simulink library "stm32f4_io_lib"  (R2015b)
settings: Solver=ode45  StartTime=0.0  StopTime=10.0  RelTol=1e-3
libraries: simulink x9
settings Model: Creator=Krisada  LastModifiedBy=Aimagin
settings DataIOCC: SaveFormat=Array  SignalLoggingSaveFormat=ModelDataLogs
settings OptimizationCC: ExpressionDepthLimit=2147483647
settings DebuggingCC: UnderspecifiedInitializationDetection=Classic  MergeDetectMultiDrivingBlocksExec=none  SolverPrmCheckMsg=warning  FcnCallInpInsideContextMsg=UseLocalSettings  StateNameClashWarn=warning  StrictBusMsg=Warning
settings HardwareCC: ProdBitPerPointer=32  ProdLargestAtomicFloat=None  ProdIntDivRoundTo=Undefined  ProdEndianess=Unspecified  ProdWordSize=32  ProdHWDeviceType=32-bit Generic
settings GRTTargetCC: CombineOutputUpdateFcns=off  GRTInterface=on
settings ConfigComp: CovModelRefEnable=Off

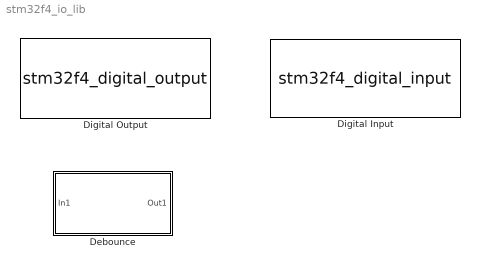
== system stm32f4_io_lib ==
  Debounce : Subsystem  TreatAsAtomicUnit=on  mask{mode=Normal, prescale=4, debounce=4}
      mask prompts: prescale "Prescale (Debounce count)"; debounce "Debounce value"
      mask help:
      | Mode,
      | 1. Normal:
      |  - Output state is 0 (FALSE) when input is steady at 0 for a Debounce period (or longer).
      |  - Output state is 1 (TRUE) when input is steady at non-zero for a Debounce period (or longer).
      |
      | 2. Single Pulse:
      |  - Output state will generate a single pulse (one time-step) when input signal change from 0-to-NonZero and steady for a Debounce period.
      |
      | 3. Toggle Latch:
      |  - Output state will toggle when input signal change from 0-to-NonZero and steady for a Debounce period
      |
      | Debounce period,
      |  - Debounce period (sec) = Debounce count * Sample time (sec)
      |
      | Note: the block is Masked Subsystem, to see its function: from the popup menu on mouse right-click, select "Look Under Mask".
      settings: RTWFcnNameOpts=Use subsystem name  RTWFileNameOpts=Use function name
      mask Help: web(fullfile(waijungdocroot,'gpio_debounce.htm'),'-browser')
      mask TypeOptions mode: Normal | Single Pulse | Toggle Latch
      mask Callback mode: waijung_intput_validation_callback('mode');
      mask TypeOptions prescale: 4 | 8 | 16 | 32 | 64 | 128 | 256 | 512 | 1024 | 2048 | 4096 | 8192
      mask Callback debounce: waijung_intput_validation_callback('prescale');
      mask Display: disp('Button Pressed\n(Normal)\nDebounce count: 4');
  Digital Input : S-Function  FunctionName=stm32f4_digital_input  Parameters=port,speed,porttype,porttypestr,use_pin0,use_pin1,use_pin2,use_pin3,use_pin4,use_pin5,use_pin6,use_pin7,use_pin8,use_pin9,use_pin10,use_pin11,use_pin12,use_pin13,use_pin14,use_pin15,pinstr,usedpinarray,bitbandingstr,sampletime,sampletimestr,blockid,glabalinit  SFunctionDeploymentMode=off  EnableBusSupport=off  mask(stm32f4_digital_input){port=A, speed=100, porttype=None, porttypestr=NOPULL, use_pin0=on, use_pin1=on, use_pin2=off, use_pin3=off, use_pin4=off, use_pin5=off, use_pin6=off, use_pin7=off, use_pin8=off, use_pin9=off, use_pin10=off, use_pin11=off, use_pin12=off, use_pin13=off, use_pin14=off, use_pin15=off, pinstr=GPIO_Pin_0 | GPIO_Pin_1, usedpinarray=[1  1  0  0  0  0  0  0  0  0  0  0  0  0  0  0], bitbandingstr=|, sampletime=-1, sampletimestr=0, blockid=DigitalInput, enablecustomportlabel=off, glabalinit=off, cinputportlabel=In1, In2, coutputportlabel=Out1, Out2}
      mask bitbandingstr=|
      | #define DigitalInput_A0 Peripheral_BB(GPIOA->IDR, 0)  /* Output pin */
      | #define DigitalInput_A1 Peripheral_BB(GPIOA->IDR, 1)  /* Output pin */
      mask prompts: speed "Speed (MHz)"; porttype "Type (Pull-Up/Pull-Down)"; porttypestr "Type (Pull Up/Pull Down) String"; use_pin0 "Use Pin 0"; use_pin1 "Use Pin 1"; use_pin2 "Use Pin 2"; use_pin3 "Use Pin 3"; use_pin4 "Use Pin 4"; use_pin5 "Use Pin 5"; use_pin6 "Use Pin 6"; use_pin7 "Use Pin 7"; use_pin8 "Use Pin 8"; use_pin9 "Use Pin 9"; use_pin10 "Use Pin 10"; use_pin11 "Use Pin 11"; use_pin12 "Use Pin 12"; use_pin13 "Use Pin 13"; use_pin14 "Use Pin 14"; use_pin15 "Use Pin 15"; pinstr "Pin string"; usedpinarray "Used pin array"; bitbandingstr "Bit banding string"; sampletime "Sample time (sec)"; sampletimestr "Compiled sample time (sec) in string"; enablecustomportlabel "Enable custom port labels"; glabalinit "Use global initialization"; cinputportlabel "Custom input port labels (Ex. In1, In2, In3)"; coutputportlabel "Custom output port labels (Ex. Out1, Out2, Out3)"
      mask help: This block implements Digital Input Module.
      mask init:
      | stm32f4_digital_input_callback('init');
      mask Help: web(fullfile(waijungdocroot,'stm32f4_digital_input.htm'), '-browser')
      mask TypeOptions port: A | B | C | D | E | F | G | H | I | J | K
      mask Callback port: stm32f4_digital_input_callback('port');
      mask TypeOptions speed: 2 | 25 | 50 | 100
      mask Callback speed: stm32f4_digital_input_callback('speed');
      mask TypeOptions porttype: None | Pull Up | Pull Down
      mask Callback porttype: stm32f4_digital_input_callback('porttype');
      mask Callback porttypestr: stm32f4_digital_input_callback('porttypestr');
      mask Callback pinstr: stm32f4_digital_input_callback('pinstr');
      mask Callback usedpinarray: stm32f4_digital_input_callback('usedpinarray');
      mask Callback bitbandingstr: stm32f4_digital_input_callback('bitbandingstr');
      mask Callback sampletime: stm32f4_digital_input_callback('sampletime');
      mask Callback sampletimestr: stm32f4_digital_input_callback('sampletimestr');
      mask Callback blockid: stm32f4_digital_input_callback('blockid');
      mask Callback enablecustomportlabel: stm32f4_digital_input_callback('enablecustomportlabel');
      mask Display: text(0.05, 0.5, 'Port: A\nSpeed (MHz): 100\nType (PU/PD): None\nTs (sec): 0','ver','middle','hor','left');port_label('output', 1,'PA0');port_label('output', 2,'PA1')
  Digital Output : S-Function  FunctionName=stm32f4_digital_output  Parameters=use_bitband,port,speed,porttype,porttypestr,use_pin0,use_pin1,use_pin2,use_pin3,use_pin4,use_pin5,use_pin6,use_pin7,use_pin8,use_pin9,use_pin10,use_pin11,use_pin12,use_pin13,use_pin14,use_pin15,pinstr,usedpinarray,bitbandingstr,sampletime,sampletimestr,blockid,globalinit  SFunctionDeploymentMode=off  EnableBusSupport=off  mask(stm32f4_digital_output){use_bitband=on, port=D, speed=100, porttype=Push Pull, porttypestr=PP, use_pin0=off, use_pin1=off, use_pin2=off, use_pin3=off, use_pin4=off, use_pin5=off, use_pin6=off, use_pin7=off, use_pin8=off, use_pin9=off, use_pin10=off, use_pin11=off, use_pin12=on, use_pin13=on, use_pin14=on, use_pin15=on, pinstr=GPIO_Pin_12 | GPIO_Pin_13 | GPIO_Pin_14 | GPIO_Pin_15, usedpinarray=[0  0  0  0  0  0  0  0  0  0  0  0  1  1  1  1], bitbandingstr=|, sampletime=-1, sampletimestr=0, blockid=DigitalOutput, enablecustomportlabel=off, globalinit=off, cinputportlabel=In1, In2, coutputportlabel=0}
      mask bitbandingstr=|
      | #define DigitalOutput_D12 Peripheral_BB(GPIOD->ODR, 12)  /* Output pin */
      | #define DigitalOutput_D13 Peripheral_BB(GPIOD->ODR, 13)  /* Output pin */
      | #define DigitalOutput_D14 Peripheral_BB(GPIOD->ODR, 14)  /* Output pin */
      | #define DigitalOutput_D15 Peripheral_BB(GPIOD->ODR, 15)  /* Output pin */
      mask prompts: use_bitband "Use Bit banding"; speed "Speed (MHz)"; porttype "Type (Push-Pull/Open-Drain)"; porttypestr "Type (Push-Pull/Open-Drain) String"; use_pin0 "Use Pin 0"; use_pin1 "Use Pin 1"; use_pin2 "Use Pin 2"; use_pin3 "Use Pin 3"; use_pin4 "Use Pin 4"; use_pin5 "Use Pin 5"; use_pin6 "Use Pin 6"; use_pin7 "Use Pin 7"; use_pin8 "Use Pin 8"; use_pin9 "Use Pin 9"; use_pin10 "Use Pin 10"; use_pin11 "Use Pin 11"; use_pin12 "Use Pin 12"; use_pin13 "Use Pin 13"; use_pin14 "Use Pin 14"; use_pin15 "Use Pin 15"; pinstr "Pin string"; usedpinarray "Used pin array"; bitbandingstr "Bit banding string"; sampletime "Sample time (sec)"; sampletimestr "Compiled sample time (sec) in string"; enablecustomportlabel "Enable custom port labels"; globalinit "Use global initialization"; cinputportlabel "Custom input port labels (Ex. In1, In2, In3)"; coutputportlabel "Custom output port labels (Ex. Out1, Out2, Out3)"
      mask help: This block implements Digital Output Module.
      mask init:
      | stm32f4_digital_output_callback('init');
      mask Help: web(fullfile(waijungdocroot,'stm32f4_digital_output.htm'),'-browser')
      mask TypeOptions port: A | B | C | D | E | F | G | H | I | J | K
      mask Callback port: stm32f4_digital_output_callback('port');
      mask TypeOptions speed: 2 | 25 | 50 | 100
      mask Callback speed: stm32f4_digital_output_callback('speed');
      mask TypeOptions porttype: Push Pull | Open Drain
      mask Callback porttype: stm32f4_digital_output_callback('porttype');
      mask Callback porttypestr: stm32f4_digital_output_callback('porttypestr');
      mask Callback pinstr: stm32f4_digital_output_callback('pinstr');
      mask Callback usedpinarray: stm32f4_digital_output_callback('usedpinarray');
      mask Callback bitbandingstr: stm32f4_digital_output_callback('bitbandingstr');
      mask Callback sampletime: stm32f4_digital_output_callback('sampletime');
      mask Callback sampletimestr: stm32f4_digital_output_callback('sampletimestr');
      mask Callback blockid: stm32f4_digital_output_callback('blockid');
      mask Callback enablecustomportlabel: stm32f4_digital_output_callback('enablecustomportlabel');
      mask Display: text(0.95, 0.5, 'Port: D\nSpeed (MHz): 100\nType (PP/OD): Push Pull\nTs (sec): 0','ver','middle','hor','right');port_label('input', 1,'PD12');port_label('input', 2,'PD13');port_label('input', 3,'PD14');port_label('input', 4,'PD15')

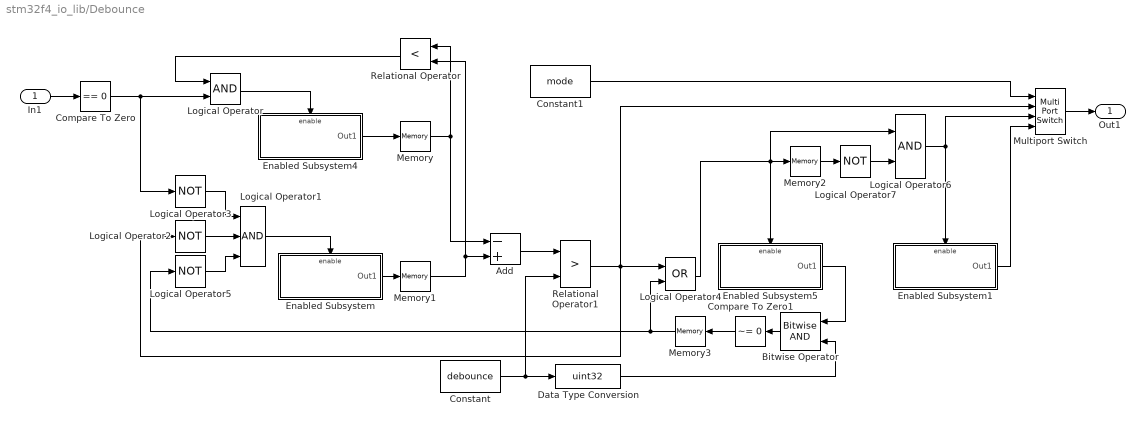
== system stm32f4_io_lib/Debounce ==
  In1 : Inport
  Add : Sum  Inputs=-+  OutDataTypeStr=int32
  Bitwise Operator : simulink/Logic and Bit Operations/Bitwise Operator  logicop=AND  UseBitMask=off  NumInputPorts=2  BitMask=debouce  BitMaskRealWorld=Stored Integer
  Compare To Zero : simulink/Logic and Bit Operations/Compare To Zero  SystemSampleTime=-1  relop===  LogicOutDataTypeMode=uint8  ZeroCross=off
  Compare To Zero1 : simulink/Logic and Bit Operations/Compare To Zero  SystemSampleTime=-1  relop=~=  LogicOutDataTypeMode=boolean  ZeroCross=off
  Constant : Constant  Value=debounce  OutDataTypeStr=int32  SampleTime=-1
  Constant1 : Constant  Value=mode  OutDataTypeStr=int32  SampleTime=-1
  Data Type Conversion : DataTypeConversion  OutDataTypeStr=uint32
  Enabled Subsystem : Subsystem  TreatAsAtomicUnit=on
  Enabled Subsystem1 : Subsystem  TreatAsAtomicUnit=on
  Enabled Subsystem4 : Subsystem  TreatAsAtomicUnit=on
  Enabled Subsystem5 : Subsystem  TreatAsAtomicUnit=on
  Logical Operator : Logic  AllPortsSameDT=off  OutDataTypeStr=boolean
  Logical Operator1 : Logic  Inputs=3  AllPortsSameDT=off  OutDataTypeStr=boolean
  Logical Operator{2..3,5,7} (4 alike) : Logic  Operator=NOT  AllPortsSameDT=off  OutDataTypeStr=boolean
  Logical Operator4 : Logic  Operator=OR  AllPortsSameDT=off  OutDataTypeStr=boolean
  Logical Operator6 : Logic  AllPortsSameDT=off  OutDataTypeStr=boolean
  Memory{,1..3} (4 alike) : Memory  InheritSampleTime=on  LinearizeMemory=on  LinearizeAsDelay=on
  Multiport Switch : MultiPortSwitch
  Relational Operator : RelationalOperator  Operator=<  OutDataTypeStr=boolean
  Relational Operator1 : RelationalOperator  Operator=>  OutDataTypeStr=boolean  InputSameDT=on
  Out1 : Outport
  wires:
  Constant1/1 -> Multiport Switch/1
  Multiport Switch/1 -> Out1/1
  Data Type Conversion/1 -> Bitwise Operator/2
  Enabled Subsystem1/1(Out1) -> Multiport Switch/4
  Logical Operator6/1 -> Enabled Subsystem1/Enable, Multiport Switch/3
  In1/1 -> Compare To Zero/1
  Enabled Subsystem/1(Out1) -> Memory1/1
  Enabled Subsystem4/1(Out1) -> Memory/1
  Memory/1 -> Relational Operator/1, Add/1
  Memory1/1 -> Add/2, Relational Operator/2
  Compare To Zero/1 -> Logical Operator/2, Logical Operator3/1
  Logical Operator/1 -> Enabled Subsystem4/Enable
  Relational Operator/1 -> Logical Operator/1
  Add/1 -> Relational Operator1/1
  Constant/1 -> Data Type Conversion/1, Relational Operator1/2
  Logical Operator2/1 -> Logical Operator1/2
  Memory3/1 -> Logical Operator4/2, Logical Operator5/1
  Logical Operator5/1 -> Logical Operator1/3
  Logical Operator3/1 -> Logical Operator1/1
  Compare To Zero1/1 -> Memory3/1
  Bitwise Operator/1 -> Compare To Zero1/1
  Enabled Subsystem5/1(Out1) -> Bitwise Operator/1
  Logical Operator4/1 -> Enabled Subsystem5/Enable, Memory2/1, Logical Operator6/1
  Memory2/1 -> Logical Operator7/1
  Logical Operator7/1 -> Logical Operator6/2
  Relational Operator1/1 -> Multiport Switch/2, Logical Operator4/1, Logical Operator2/1
  Logical Operator1/1 -> Enabled Subsystem/Enable

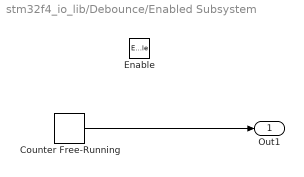
== system stm32f4_io_lib/Debounce/Enabled Subsystem ==
  Enable : EnablePort  PropagateVarSize=During execution
  Counter Free-Running : simulink/Sources/Counter Free-Running  SystemSampleTime=-1  NumBits=32  tsamp=-1
  Out1 : Outport  InitialOutput=0
  wires:
  Counter Free-Running/1 -> Out1/1

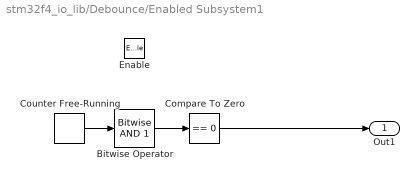
== system stm32f4_io_lib/Debounce/Enabled Subsystem1 ==
  Enable : EnablePort  PropagateVarSize=During execution
  Bitwise Operator : simulink/Logic and Bit Operations/Bitwise Operator  logicop=AND  UseBitMask=on  BitMask=1  BitMaskRealWorld=Stored Integer
  Compare To Zero : simulink/Logic and Bit Operations/Compare To Zero  SystemSampleTime=-1  relop===  LogicOutDataTypeMode=uint8  ZeroCross=off
  Counter Free-Running : simulink/Sources/Counter Free-Running  SystemSampleTime=-1  NumBits=32  tsamp=-1
  Out1 : Outport  InitialOutput=0
  wires:
  Counter Free-Running/1 -> Bitwise Operator/1
  Bitwise Operator/1 -> Compare To Zero/1
  Compare To Zero/1 -> Out1/1

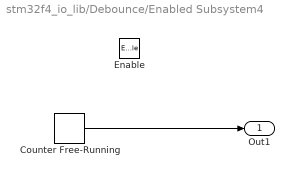
== system stm32f4_io_lib/Debounce/Enabled Subsystem4 ==
  Enable : EnablePort  PropagateVarSize=During execution
  Counter Free-Running : simulink/Sources/Counter Free-Running  SystemSampleTime=-1  NumBits=32  tsamp=-1
  Out1 : Outport  InitialOutput=0
  wires:
  Counter Free-Running/1 -> Out1/1

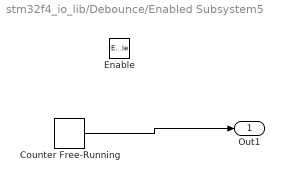
== system stm32f4_io_lib/Debounce/Enabled Subsystem5 ==
  Enable : EnablePort  PropagateVarSize=During execution
  Counter Free-Running : simulink/Sources/Counter Free-Running  SystemSampleTime=-1  NumBits=32  tsamp=-1
  Out1 : Outport  InitialOutput=0
  wires:
  Counter Free-Running/1 -> Out1/1
